simulink subsystem "rss_motor_model"  (R2022b)
settings: Solver=VariableStepAuto  StartTime=0.0  StopTime=10.0  RelTol=1e-3
settings Model: Creator=CAV2OFO  LastModifiedBy=CAV2OFO
settings SolverCC: AlgebraicLoopSolver=TrustRegion
settings DebuggingCC: UnconnectedInputMsg=warning  UnconnectedOutputMsg=warning  UnconnectedLineMsg=warning  SFMachineParentedDataDiag=warning
settings ModelReferenceCC: EnableRefExpFcnMdlSchedulingChecks=on
settings RTWCC: DLArmComputeVersion=19.05

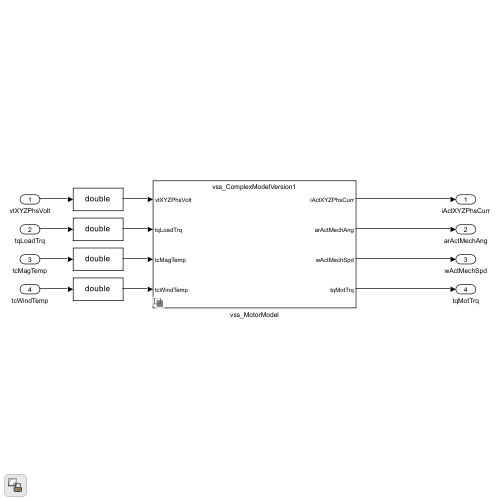
[thumbnail: Simulink's stored preview of the top-level diagram]
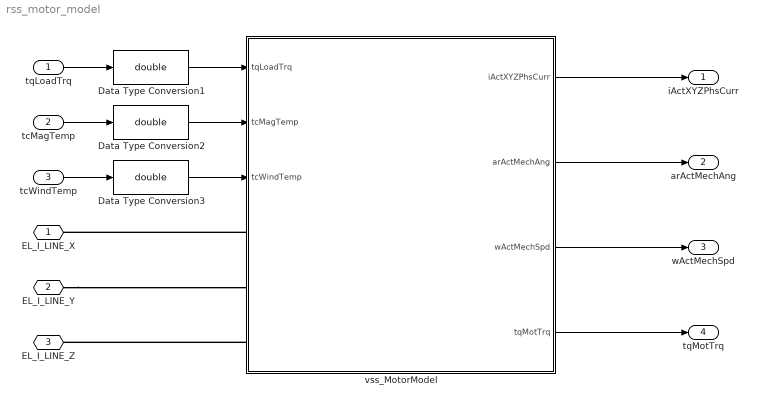
== system rss_motor_model ==
  tqLoadTrq : Inport
  tcMagTemp : Inport  Port=2
  tcWindTemp : Inport  Port=3
  Data Type Conversion1 : DataTypeConversion  OutDataTypeStr=double  SaturateOnIntegerOverflow=off  RndMeth=Floor
  Data Type Conversion2 : DataTypeConversion  OutDataTypeStr=double  SaturateOnIntegerOverflow=off  RndMeth=Floor
  Data Type Conversion3 : DataTypeConversion  OutDataTypeStr=double  SaturateOnIntegerOverflow=off  RndMeth=Floor
  vss_MotorModel : Subsystem  Variant=on
  EL_I_LINE_X : PMIOPort  Side=Left
  EL_I_LINE_Y : PMIOPort  Port=2  Side=Left
  EL_I_LINE_Z : PMIOPort  Port=3  Side=Left
  iActXYZPhsCurr : Outport
  arActMechAng : Outport  Port=2
  wActMechSpd : Outport  Port=3
  tqMotTrq : Outport  Port=4
  wires:
  vss_MotorModel/3(wActMechSpd) -> wActMechSpd/1
  vss_MotorModel/1(iActXYZPhsCurr) -> iActXYZPhsCurr/1
  vss_MotorModel/2(arActMechAng) -> arActMechAng/1
  tqLoadTrq/1 -> Data Type Conversion1/1
  vss_MotorModel/4(tqMotTrq) -> tqMotTrq/1
  tcMagTemp/1 -> Data Type Conversion2/1
  tcWindTemp/1 -> Data Type Conversion3/1
  Data Type Conversion1/1 -> vss_MotorModel/1(tqLoadTrq)
  Data Type Conversion3/1 -> vss_MotorModel/3(tcWindTemp)
  Data Type Conversion2/1 -> vss_MotorModel/2(tcMagTemp)
  connections:
  vss_MotorModel/LConn1 -- EL_I_LINE_X/RConn1
  EL_I_LINE_Y/RConn1 -- vss_MotorModel/LConn2
  vss_MotorModel/LConn3 -- EL_I_LINE_Z/RConn1

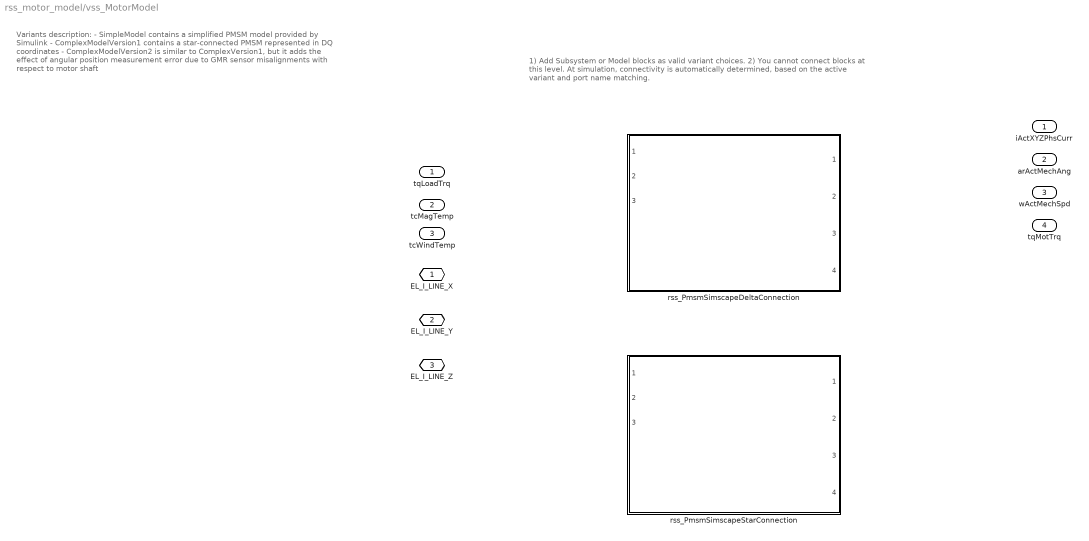
== system rss_motor_model/vss_MotorModel ==
  note: 1) Add Subsystem or Model blocks as valid variant choices.
      | 2) You cannot connect blocks at this level. At simulation, connectivity is automatically
      | determined, based on the active variant and port name matching.
  note: Variants description:
      | - SimpleModel contains a simplified PMSM model provided by Simulink
      | - ComplexModelVersion1 contains a star-connected PMSM represented
      | in DQ coordinates
      | - ComplexModelVersion2 is similar to ComplexVersion1, but it adds the
      | effect of angular position measurement error due to GMR sensor misalignments
      | with respect to motor shaft
  tqLoadTrq : Inport  OutDataTypeStr=double
  tcMagTemp : Inport  Port=2  OutDataTypeStr=double
  tcWindTemp : Inport  Port=3  OutDataTypeStr=double
  rss_PmsmSimscapeDeltaConnection : Subsystem  VariantControl=parMotType == MOT_TYPE.DELTA  ReferencedSubsystem=rss_pmsm_motor_simscape_deltaconn
  rss_PmsmSimscapeStarConnection : Subsystem  VariantControl=parMotType == MOT_TYPE.STAR  ReferencedSubsystem=rss_pmsm_motor_simscape_starconn
  EL_I_LINE_X : PMIOPort  Side=Left
  EL_I_LINE_Y : PMIOPort  Port=2  Side=Left
  EL_I_LINE_Z : PMIOPort  Port=3  Side=Left
  iActXYZPhsCurr : Outport
  arActMechAng : Outport  Port=2
  wActMechSpd : Outport  Port=3
  tqMotTrq : Outport  Port=4
